simulink model "sampleModel1757"  (R2023a)
settings: Solver=VariableStepAuto  StartTime=0.0  StopTime=10.0  RelTol=1e-3
libraries: hdlsllib x6, simulink x4
settings Model: Creator=user1  LastModifiedBy=user1

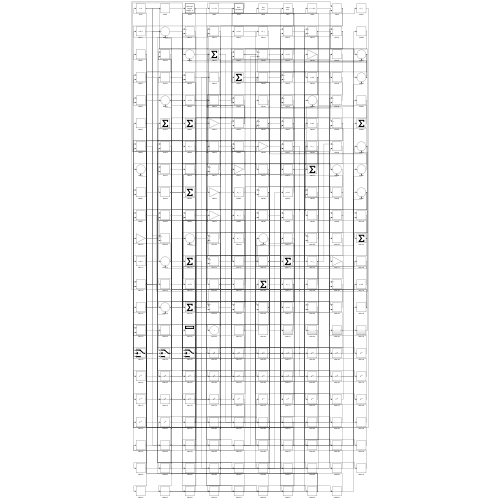
[thumbnail: Simulink's stored preview of the top-level diagram]
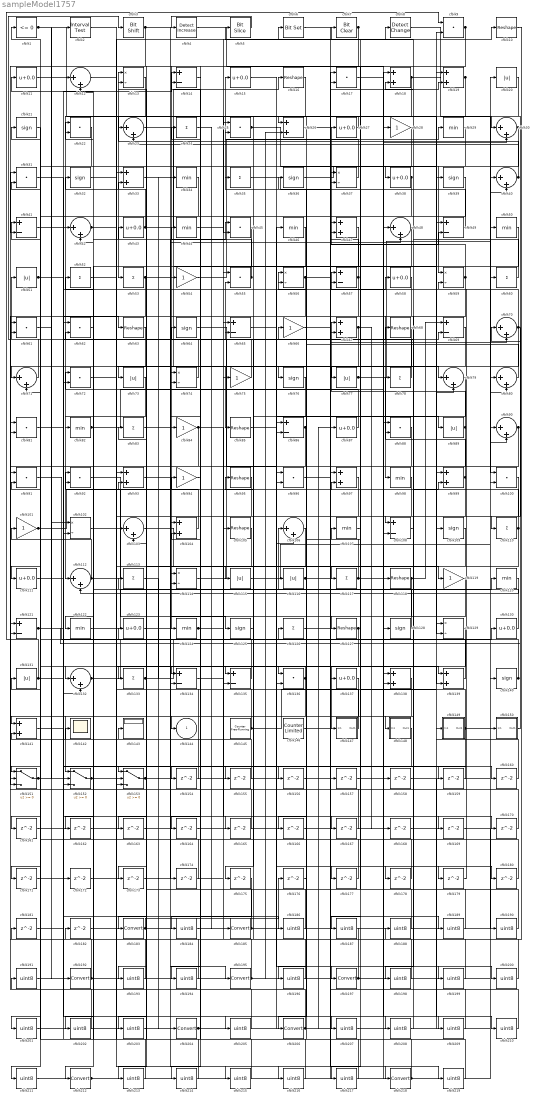
== system sampleModel1757 ==
  cfblk1 : hdlsllib/Logic and Bit Operations/Compare To Zero  relop=<=  OutDataTypeStr=boolean
  cfblk{10,16,63,68,85,95,105,118,127} (9 alike) : Reshape
  cfblk{9,17,22,25,31,45,55,61..62,72,81,88,91..92,96,100,136} (17 alike) : DotProduct  OutDataTypeStr=Inherit: Inherit via internal rule
  cfblk{28,54,66,75,84,94,101,119} (8 alike) : Gain
  cfblk{13,37,56,59,74,102,114,129} (8 alike) : Product  Inputs=*/  RndMeth=Zero  SaturateOnIntegerOverflow=on
  cfblk{12,23,30,40,42,48,70..71,79..80,90,103,106,112,132} (15 alike) : Sum  Inputs=|++
  cfblk{18..19,26,33,47,67,93,97,99,104,138..139,141} (13 alike) : Sum
  cfblk{29,34,44,46,50,82,98,107,120,122,124} (11 alike) : MinMax
  cfblk{14,41,49,57,65,69,86,108,121,134..135} (11 alike) : Sum  Inputs=+-
  cfblk{21,32,36,39,64,76,109,125,128,140} (10 alike) : Signum
  cfblk{11,15,27,38,43,58,87,111,123,130,137} (11 alike) : Bias  Bias=0.0  SaturateOnIntegerOverflow=off
  cfblk{24,35,52..53,60,78,83,110,113,117,126,133} (12 alike) : Sum  Inputs=+
  cfblk{20,51,73,77,89,115..116,131} (8 alike) : Abs  SaturateOnIntegerOverflow=off
  cfblk142 : Scope
  cfblk143 : Display
  cfblk145 : hdlsllib/Sources/Counter Free-Running  NumBits=16  tsamp=-1
  cfblk146 : hdlsllib/Sources/Counter Limited  uplimit=7  tsamp=-1
  cfblk147 : Subsystem
      settings: LibrarySourceBlock=|
      | hdlsllib/Ports &
      | Subsystems/Subsystem
  cfblk148 : Subsystem
      settings: LibrarySourceBlock=|
      | hdlsllib/Ports &
      | Subsystems/Subsystem
  cfblk149 : Subsystem
      settings: LibrarySourceBlock=|
      | hdlsllib/Ports &
      | Subsystems/Subsystem
  cfblk150 : Subsystem
      settings: LibrarySourceBlock=|
      | hdlsllib/Ports &
      | Subsystems/Subsystem
  cfblk151 : Switch  SaturateOnIntegerOverflow=off  InputSameDT=off
  cfblk152 : Switch  SaturateOnIntegerOverflow=off  InputSameDT=off
  cfblk153 : Switch  SaturateOnIntegerOverflow=off  InputSameDT=off
  cfblk{154..182} (29 alike) : Delay  SampleTime=1
  cfblk{183,185,192,195,197,204,206,212,218} (9 alike) : DataTypeConversion  SaturateOnIntegerOverflow=off  RndMeth=Floor
  cfblk{184,186..191,193..194,196,198..203,205,207..211,213..217,219} (28 alike) : DataTypeConversion  OutDataTypeStr=uint8  SaturateOnIntegerOverflow=off  RndMeth=Floor
  cfblk2 : hdlsllib/Logic and Bit Operations/Interval Test  IntervalClosedRight=on  uplimit=0.5  IntervalClosedLeft=on  lowlimit=-0.5  OutDataTypeStr=boolean
  cfblk3 : hdlsllib/Logic and Bit Operations/Bit Shift  mode=Shift Left Logical  N=0
  cfblk4 : simulink/Logic and Bit Operations/Detect Increase  vinit=0.0  OutDataTypeStr=boolean
      settings: LibrarySourceBlock=|
      | hdlsllib/Logic and Bit
      | Operations/Detect
      | Increase
  cfblk5 : hdlsllib/Logic and Bit Operations/Bit Slice  lidx=7  ridx=0
  cfblk6 : simulink/Logic and Bit Operations/Bit Set  iBit=0
      settings: LibrarySourceBlock=|
      | hdlsllib/Logic and Bit
      | Operations/Bit Set
  cfblk7 : simulink/Logic and Bit Operations/Bit Clear  iBit=0
      settings: LibrarySourceBlock=|
      | hdlsllib/Logic and Bit
      | Operations/Bit Clear
  cfblk8 : simulink/Logic and Bit Operations/Detect Change  vinit=0  OutDataTypeStr=boolean
      settings: LibrarySourceBlock=|
      | hdlsllib/Logic and Bit
      | Operations/Detect
      | Change
  cfblk144 : Outport  VectorParamsAs1DForOutWhenUnconnected=off
  wires:
  cfblk13/1 -> cfblk112/1
  cfblk89/1 -> cfblk67/1, cfblk133/1
  cfblk130/1 -> cfblk52/1
  cfblk54/1 -> cfblk29/1
  cfblk92/1 -> cfblk125/1
  cfblk128/1 -> cfblk106/1
  cfblk30/1 -> cfblk59/1, cfblk23/2
  cfblk91/1 -> cfblk130/1
  cfblk121/1 -> cfblk30/1, cfblk2/1, cfblk69/2, cfblk207/1
  cfblk40/1 -> cfblk13/1, cfblk14/1
  cfblk114/1 -> cfblk66/1
  cfblk150/1(Out1) -> cfblk70/1
  cfblk9/1 -> cfblk124/1, cfblk217/1
  cfblk49/1 -> cfblk15/1
  cfblk57/1 -> cfblk27/1, cfblk153/1, cfblk81/2
  cfblk7/1 -> cfblk73/1, cfblk144/1
  cfblk65/1 -> cfblk197/1
  cfblk120/1 -> cfblk112/2
  cfblk24/1 -> cfblk185/1
  cfblk145/1 -> cfblk13/2, cfblk19/1
  cfblk43/1 -> cfblk16/1, cfblk109/1, cfblk12/2
  cfblk41/1 -> cfblk42/1
  cfblk140/1 -> cfblk32/1, cfblk104/2
  cfblk38/1 -> cfblk104/1, cfblk138/2
  cfblk112/1 -> cfblk94/1, cfblk41/1
  cfblk73/1 -> cfblk82/1
  cfblk50/1 -> cfblk77/1
  cfblk15/1 -> cfblk106/2
  cfblk36/1 -> cfblk38/1
  cfblk136/1 -> cfblk132/1, cfblk151/2
  cfblk29/1 -> cfblk86/2
  cfblk133/1 -> cfblk80/1, cfblk34/1
  cfblk115/1 -> cfblk60/1
  cfblk86/1 -> cfblk136/1, cfblk175/1
  cfblk122/1 -> cfblk120/1
  cfblk39/1 -> cfblk74/1
  cfblk83/1 -> cfblk195/1
  cfblk55/1 -> cfblk11/1, cfblk44/1
  cfblk82/1 -> cfblk67/2, cfblk28/1, cfblk216/1
  cfblk118/1 -> cfblk69/1, cfblk184/1
  cfblk125/1 -> cfblk95/1
  cfblk135/1 -> cfblk22/1
  cfblk103/1 -> cfblk117/1
  cfblk16/1 -> cfblk135/1
  cfblk113/1 -> cfblk204/1
  cfblk71/1 -> cfblk3/1
  cfblk4/1 -> cfblk118/1
  cfblk117/1 -> cfblk35/1, cfblk30/2
  cfblk151/1 -> cfblk12/1, cfblk205/1, cfblk208/1
  cfblk23/1 -> cfblk76/1
  cfblk64/1 -> cfblk116/1
  cfblk28/1 -> cfblk111/1
  cfblk61/1 -> cfblk192/1
  cfblk138/1 -> cfblk152/1
  cfblk20/1 -> cfblk53/1
  cfblk109/1 -> cfblk134/1
  cfblk68/1 -> cfblk127/1
  cfblk2/1 -> cfblk139/1
  cfblk127/1 -> cfblk161/1, cfblk162/1
  cfblk124/1 -> cfblk136/2, cfblk97/2
  cfblk131/1 -> cfblk9/1, cfblk14/2, cfblk57/2
  cfblk102/1 -> cfblk139/2
  cfblk70/1 -> cfblk110/1, cfblk57/1, cfblk196/1
  cfblk105/1 -> cfblk183/1
  cfblk129/1 -> cfblk147/1(In1)
  cfblk69/1 -> cfblk85/1
  cfblk149/1(Out1) -> cfblk7/1, cfblk90/2, cfblk214/1
  cfblk78/1 -> cfblk51/1
  cfblk5/1 -> cfblk4/1
  cfblk110/1 -> cfblk18/2, cfblk155/1
  cfblk123/1 -> cfblk54/1
  cfblk152/1 -> cfblk92/1, cfblk10/1
  cfblk42/1 -> cfblk79/1, cfblk165/1
  cfblk53/1 -> cfblk45/1, cfblk102/2
  cfblk132/1 -> cfblk18/1, cfblk99/2
  cfblk75/1 -> cfblk55/2
  cfblk77/1 -> cfblk20/1, cfblk137/1
  cfblk134/1 -> cfblk58/1
  cfblk116/1 -> cfblk49/2, cfblk170/1
  cfblk34/1 -> cfblk151/1
  cfblk97/1 -> cfblk114/1
  cfblk87/1 -> cfblk42/2
  cfblk19/1 -> cfblk45/2, cfblk47/2
  cfblk146/1 -> cfblk70/2
  cfblk139/1 -> cfblk91/2
  cfblk88/1 -> cfblk206/1
  cfblk100/1 -> cfblk148/1(In1)
  cfblk67/1 -> cfblk72/2, cfblk168/1
  cfblk60/1 -> cfblk5/1
  cfblk58/1 -> cfblk98/1
  cfblk1/1 -> cfblk39/1, cfblk102/1
  cfblk52/1 -> cfblk8/1
  cfblk84/1 -> cfblk151/3, cfblk167/1
  cfblk80/1 -> cfblk56/1
  cfblk47/1 -> cfblk114/2
  cfblk147/1(Out1) -> cfblk43/1
  cfblk74/1 -> cfblk33/2
  cfblk8/1 -> cfblk40/1
  cfblk62/1 -> cfblk212/1
  cfblk59/1 -> cfblk141/1, cfblk47/1, cfblk198/1
  cfblk90/1 -> cfblk122/1, cfblk171/1
  cfblk22/1 -> cfblk71/1
  cfblk101/1 -> cfblk75/1, cfblk132/2
  cfblk37/1 -> cfblk25/2
  cfblk12/1 -> cfblk119/1
  cfblk14/1 -> cfblk84/1
  cfblk31/1 -> cfblk63/1
  cfblk51/1 -> cfblk21/1, cfblk160/1
  cfblk95/1 -> cfblk103/2
  cfblk56/1 -> cfblk121/2, cfblk19/2
  cfblk35/1 -> cfblk37/2
  cfblk44/1 -> cfblk6/1
  cfblk3/1 -> cfblk48/2, cfblk41/2
  cfblk99/1 -> cfblk78/1, cfblk153/3
  cfblk104/1 -> cfblk72/1
  cfblk27/1 -> cfblk26/1
  cfblk98/1 -> cfblk108/1
  cfblk18/1 -> cfblk100/1, cfblk156/1
  cfblk153/1 -> cfblk108/2, cfblk50/1, cfblk174/1
  cfblk126/1 -> cfblk218/1
  cfblk108/1 -> cfblk68/1
  cfblk25/1 -> cfblk129/2, cfblk89/1
  cfblk119/1 -> cfblk134/2
  cfblk76/1 -> cfblk115/1
  cfblk11/1 -> cfblk23/1
  cfblk72/1 -> cfblk154/1
  cfblk154/1 -> cfblk33/1
  cfblk155/1 -> cfblk121/1
  cfblk32/1 -> cfblk159/1
  cfblk159/1 -> cfblk152/2
  cfblk160/1 -> cfblk99/1
  cfblk161/1 -> cfblk103/1
  cfblk162/1 -> cfblk135/2
  cfblk45/1 -> cfblk163/1
  cfblk163/1 -> cfblk86/1
  cfblk94/1 -> cfblk164/1
  cfblk164/1 -> cfblk48/1
  cfblk165/1 -> cfblk91/1
  cfblk79/1 -> cfblk166/1
  cfblk166/1 -> cfblk40/2
  cfblk167/1 -> cfblk92/2
  cfblk168/1 -> cfblk129/1
  cfblk111/1 -> cfblk169/1
  cfblk170/1 -> cfblk22/2
  cfblk171/1 -> cfblk153/2
  cfblk81/1 -> cfblk172/1
  cfblk172/1 -> cfblk25/1
  cfblk137/1 -> cfblk173/1
  cfblk173/1 -> cfblk74/2
  cfblk174/1 -> cfblk71/2
  cfblk176/1 -> cfblk56/2
  cfblk85/1 -> cfblk177/1
  cfblk177/1 -> cfblk55/1
  cfblk6/1 -> cfblk178/1
  cfblk178/1 -> cfblk37/1
  cfblk26/1 -> cfblk179/1
  cfblk179/1 -> cfblk59/2
  cfblk66/1 -> cfblk180/1
  cfblk180/1 -> cfblk1/1
  cfblk181/1 -> cfblk152/3
  cfblk182/1 -> cfblk138/1
  cfblk183/1 -> cfblk176/1, cfblk90/1, cfblk123/1
  cfblk184/1 -> cfblk105/1
  cfblk185/1 -> cfblk79/2, cfblk143/1
  cfblk141/1 -> cfblk186/1
  cfblk186/1 -> cfblk24/1
  cfblk107/1 -> cfblk187/1
  cfblk187/1 -> cfblk182/1
  cfblk10/1 -> cfblk188/1
  cfblk188/1 -> cfblk107/1
  cfblk96/1 -> cfblk189/1
  cfblk189/1 -> cfblk36/1
  cfblk169/1 -> cfblk190/1
  cfblk190/1 -> cfblk96/1
  cfblk191/1 -> cfblk96/2
  cfblk192/1 -> cfblk131/1, cfblk80/2
  cfblk48/1 -> cfblk193/1
  cfblk193/1 -> cfblk61/1
  cfblk175/1 -> cfblk194/1
  cfblk194/1 -> cfblk61/2
  cfblk195/1 -> cfblk9/2, cfblk26/2, cfblk101/1
  cfblk196/1 -> cfblk83/1
  cfblk197/1 -> cfblk181/1, cfblk142/1, cfblk150/1(In1)
  cfblk198/1 -> cfblk65/1
  cfblk156/1 -> cfblk199/1
  cfblk199/1 -> cfblk65/2
  cfblk157/1 -> cfblk200/1
  cfblk200/1 -> cfblk31/1
  cfblk63/1 -> cfblk201/1
  cfblk201/1 -> cfblk157/1
  cfblk46/1 -> cfblk202/1
  cfblk202/1 -> cfblk31/2
  cfblk148/1(Out1) -> cfblk203/1
  cfblk203/1 -> cfblk46/1
  cfblk204/1 -> cfblk100/2, cfblk128/1
  cfblk205/1 -> cfblk113/1
  cfblk206/1 -> cfblk81/1, cfblk149/1(In1), cfblk87/1
  cfblk207/1 -> cfblk88/1
  cfblk208/1 -> cfblk88/2
  cfblk17/1 -> cfblk209/1
  cfblk209/1 -> cfblk49/1
  cfblk158/1 -> cfblk210/1
  cfblk210/1 -> cfblk17/1
  cfblk21/1 -> cfblk211/1
  cfblk211/1 -> cfblk17/2
  cfblk212/1 -> cfblk158/1, cfblk140/1
  cfblk106/1 -> cfblk213/1
  cfblk213/1 -> cfblk62/1
  cfblk214/1 -> cfblk62/2
  cfblk93/1 -> cfblk215/1
  cfblk215/1 -> cfblk64/1
  cfblk216/1 -> cfblk93/1
  cfblk217/1 -> cfblk93/2
  cfblk218/1 -> cfblk191/1, cfblk141/2, cfblk97/1
  cfblk33/1 -> cfblk219/1
  cfblk219/1 -> cfblk126/1

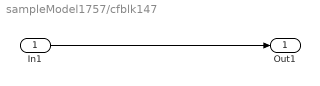
== system sampleModel1757/cfblk147 ==
  In1 : Inport
  Out1 : Outport
  wires:
  In1/1 -> Out1/1

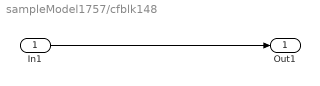
== system sampleModel1757/cfblk148 ==
  In1 : Inport
  Out1 : Outport
  wires:
  In1/1 -> Out1/1

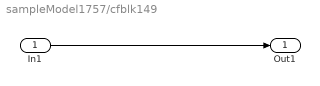
== system sampleModel1757/cfblk149 ==
  In1 : Inport
  Out1 : Outport
  wires:
  In1/1 -> Out1/1

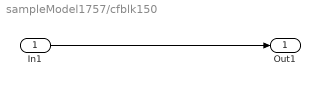
== system sampleModel1757/cfblk150 ==
  In1 : Inport
  Out1 : Outport
  wires:
  In1/1 -> Out1/1
